simulink model "ej1c"  (R2021a)
settings: Solver=VariableStepAuto  StartTime=0.0  StopTime=4  RelTol=1e-3
values from neighbouring files (symbols this model uses):
  Bm = 2*rand    [codigo.m]
  JL = 10    [codigo.m]
  Jm = 1    [codigo.m]
  KL = 500    [codigo.m]
  Km = 10    [codigo.m]
  Ra = 1    [codigo.m]
settings Model: Creator=34622  LastModifiedBy=34622

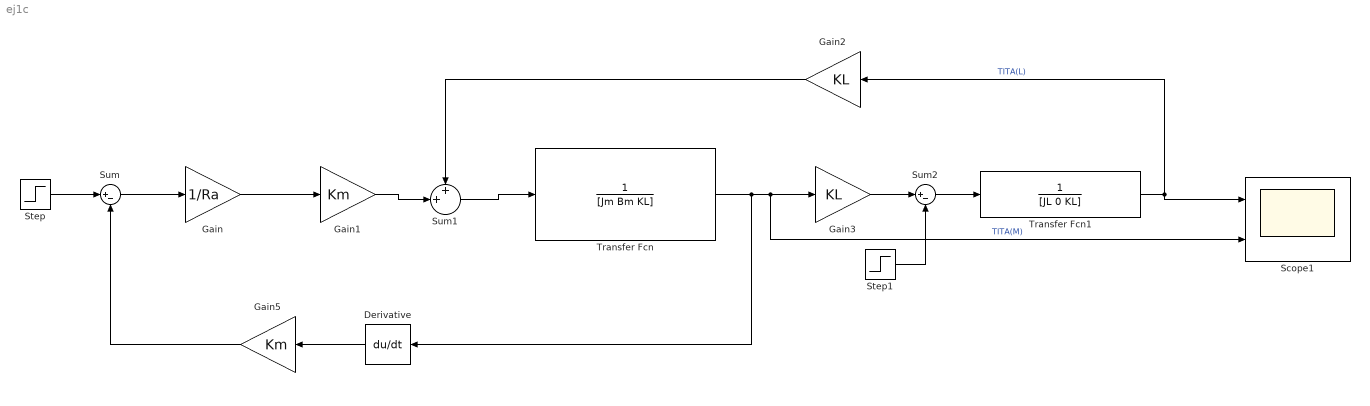
== system ej1c ==
  Derivative : Derivative
  Gain : Gain  Gain=1/Ra
  Gain1 : Gain  Gain=Km
  Gain2 : Gain  Gain=KL
  Gain3 : Gain  Gain=KL
  Gain5 : Gain  Gain=Km
  Scope1 : Scope  NumInputPorts=2
  Step : Step  Time=0  SampleTime=0
  Step1 : Step  Time=0  After=0  SampleTime=0
  Sum : Sum  Inputs=|+-
  Sum1 : Sum  Inputs=++|
  Sum2 : Sum  Inputs=|+-
  Transfer Fcn : TransferFcn  Denominator=[Jm Bm KL]
  Transfer Fcn1 : TransferFcn  Denominator=[JL 0 KL]
  wires:
  Sum/1 -> Gain/1
  Gain/1 -> Gain1/1
  Gain5/1 -> Sum/2
  Derivative/1 -> Gain5/1
  Sum1/1 -> Transfer Fcn/1
  Transfer Fcn/1 -> Derivative/1, Scope1/2, Gain3/1  "TITA(M)"
  Gain3/1 -> Sum2/1
  Sum2/1 -> Transfer Fcn1/1
  Step/1 -> Sum/1
  Step1/1 -> Sum2/2
  Gain1/1 -> Sum1/2
  Gain2/1 -> Sum1/1
  Transfer Fcn1/1 -> Scope1/1, Gain2/1  "TITA(L)"
